simulink model "UserFunctions"  (R2017b)
settings: Solver=VariableStepAuto  StartTime=0.0  StopTime=10.0  RelTol=1e-3
InitFcn:
  | InitModel
settings Model: Creator=jim  LastModifiedBy=jim

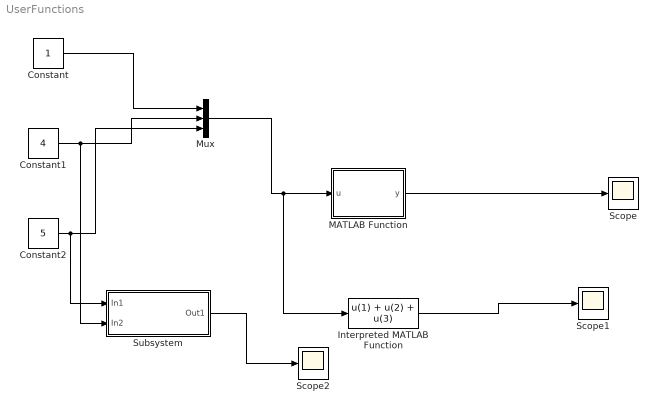
== system UserFunctions ==
  Constant : Constant
  Constant1 : Constant  Value=4
  Constant2 : Constant  Value=5
  Interpreted MATLAB Function : MATLABFcn  MATLABFcn=u(1) + u(2) + u(3)
  MATLAB Function : MATLAB Function  TreatAsAtomicUnit=on
  Mux : Mux  Inputs=3
  Scope : Scope
  Scope1 : Scope
  Scope2 : Scope
  Subsystem : Subsystem
  wires:
  MATLAB Function/1(y) -> Scope/1
  Constant/1 -> Mux/1
  Constant1/1 -> Subsystem/2(In2), Mux/2
  Constant2/1 -> Subsystem/1(In1), Mux/3
  Mux/1 -> Interpreted MATLAB Function/1, MATLAB Function/1(u)
  Interpreted MATLAB Function/1 -> Scope1/1
  Subsystem/1(Out1) -> Scope2/1

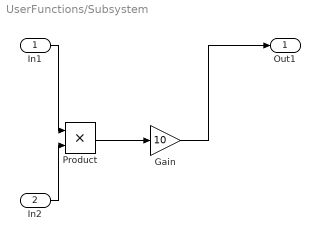
== system UserFunctions/Subsystem ==
  In1 : Inport
  In2 : Inport  Port=2
  Gain : Gain  Gain=10
  Product : Product
  Out1 : Outport
  wires:
  Gain/1 -> Out1/1
  In1/1 -> Product/1
  In2/1 -> Product/2
  Product/1 -> Gain/1

== matlab function UserFunctions/MATLAB Function ==
  data: u input; y output
function y = fcn(u)

y = u(1)+u(2)+u(3);
end
